simulink model "sampleModel1735"  (R2023a)
settings: Solver=VariableStepAuto  StartTime=0.0  StopTime=10.0  RelTol=1e-3
libraries: hdlsllib x7, simulink x2
settings Model: Creator=user1  LastModifiedBy=user1

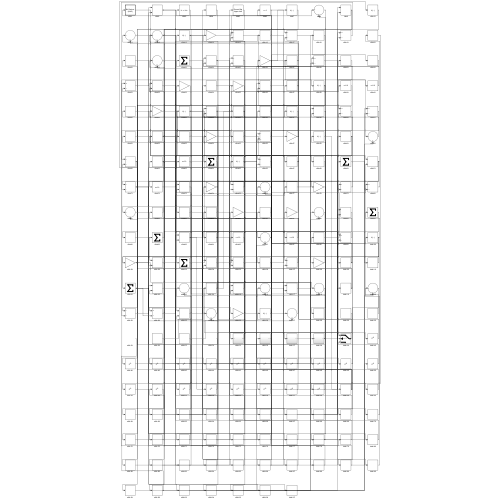
[thumbnail: Simulink's stored preview of the top-level diagram]
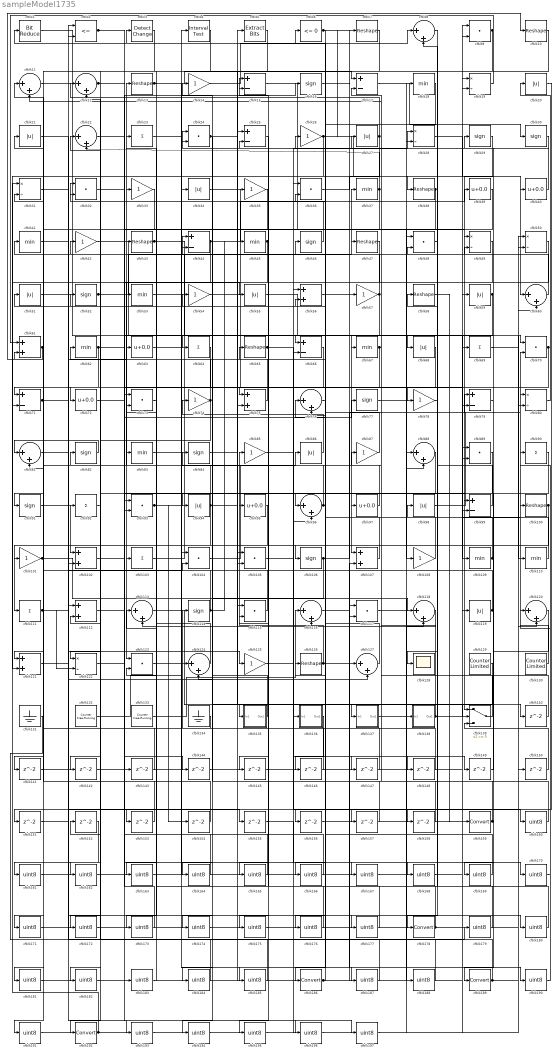
== system sampleModel1735 ==
  cfblk1 : hdlsllib/Logic and Bit Operations/Bit Reduce  mode=AND
  cfblk{7,10,13,38,43,47,58,65,100,126} (10 alike) : Reshape
  cfblk{14,26,33,35,42,54,57,74,78,85,87,101,108,125} (14 alike) : Gain
  cfblk{56,61,75,102,107,112,121} (7 alike) : Sum
  cfblk{23,64,69,90,92,103,111} (7 alike) : Sum  Inputs=+
  cfblk{9,24,32,36,48,70,73,89,93,104..105,115,117,123} (14 alike) : DotProduct  OutDataTypeStr=Inherit: Inherit via internal rule
  cfblk{16,29..30,46,52,77,82,84,91,106,114} (11 alike) : Signum
  cfblk{18,37,41,45,53,62,67,83,109..110} (10 alike) : MinMax
  cfblk{8,11..12,22,60,76,81,88,96,113,116,118,120,124,127} (15 alike) : Sum  Inputs=|++
  cfblk{20..21,27,34,51,55,59,68,86,94,98,119} (12 alike) : Abs  SaturateOnIntegerOverflow=off
  cfblk{19,28,31,49..50,80,122} (7 alike) : Product  Inputs=*/  RndMeth=Zero  SaturateOnIntegerOverflow=on
  cfblk128 : Scope
  cfblk129 : hdlsllib/Sources/Counter Limited  uplimit=7  tsamp=-1
  cfblk130 : hdlsllib/Sources/Counter Limited  uplimit=7  tsamp=-1
  cfblk131 : Ground
  cfblk132 : hdlsllib/Sources/Counter Free-Running  NumBits=16  tsamp=-1
  cfblk133 : hdlsllib/Sources/Counter Free-Running  NumBits=16  tsamp=-1
  cfblk134 : Ground
  cfblk135 : Subsystem
      settings: LibrarySourceBlock=|
      | hdlsllib/Ports &
      | Subsystems/Subsystem
  cfblk136 : Subsystem
      settings: LibrarySourceBlock=|
      | hdlsllib/Ports &
      | Subsystems/Subsystem
  cfblk137 : Subsystem
      settings: LibrarySourceBlock=|
      | hdlsllib/Ports &
      | Subsystems/Subsystem
  cfblk138 : Subsystem
      settings: LibrarySourceBlock=|
      | hdlsllib/Ports &
      | Subsystems/Subsystem
  cfblk139 : Switch  SaturateOnIntegerOverflow=off  InputSameDT=off
  cfblk{140..158} (19 alike) : Delay  SampleTime=1
  cfblk{15,17,25,44,66,71,79,99} (8 alike) : Sum  Inputs=+-
  cfblk{159,178,186,189,192} (5 alike) : DataTypeConversion  SaturateOnIntegerOverflow=off  RndMeth=Floor
  cfblk{160..177,179..185,187..188,190..191,193..197} (34 alike) : DataTypeConversion  OutDataTypeStr=uint8  SaturateOnIntegerOverflow=off  RndMeth=Floor
  cfblk2 : RelationalOperator  Operator=<=  OutDataTypeStr=boolean  InputSameDT=off
  cfblk3 : simulink/Logic and Bit Operations/Detect Change  vinit=0  OutDataTypeStr=boolean
      settings: LibrarySourceBlock=|
      | hdlsllib/Logic and Bit
      | Operations/Detect
      | Change
  cfblk{39..40,63,72,95,97} (6 alike) : Bias  Bias=0.0  SaturateOnIntegerOverflow=off
  cfblk4 : hdlsllib/Logic and Bit Operations/Interval Test  IntervalClosedRight=on  uplimit=0.5  IntervalClosedLeft=on  lowlimit=-0.5  OutDataTypeStr=boolean
  cfblk5 : simulink/Logic and Bit Operations/Extract Bits  bitsToExtract=Upper half  numBits=8  bitIdxRange=[0 7]  outScalingMode=Preserve fixed-point scaling
      settings: LibrarySourceBlock=|
      | hdlsllib/Logic and Bit
      | Operations/Extract Bits
  cfblk6 : hdlsllib/Logic and Bit Operations/Compare To Zero  relop=<=  OutDataTypeStr=boolean
  wires:
  cfblk29/1 -> cfblk139/1
  cfblk34/1 -> cfblk66/1
  cfblk127/1 -> cfblk3/1
  cfblk57/1 -> cfblk37/1, cfblk124/2, cfblk14/1
  cfblk113/1 -> cfblk137/1(In1)
  cfblk82/1 -> cfblk81/1
  cfblk60/1 -> cfblk41/1
  cfblk103/1 -> cfblk46/1
  cfblk15/1 -> cfblk108/1
  cfblk126/1 -> cfblk85/1, cfblk148/1
  cfblk134/1 -> cfblk114/1
  cfblk108/1 -> cfblk82/1
  cfblk43/1 -> cfblk70/1, cfblk117/2
  cfblk109/1 -> cfblk62/1, cfblk8/2
  cfblk74/1 -> cfblk122/1, cfblk12/2
  cfblk130/1 -> cfblk70/2
  cfblk107/1 -> cfblk51/1
  cfblk53/1 -> cfblk124/1
  cfblk96/1 -> cfblk11/1, cfblk56/2
  cfblk64/1 -> cfblk123/1
  cfblk26/1 -> cfblk60/1, cfblk71/2, cfblk7/1
  cfblk123/1 -> cfblk104/1
  cfblk97/1 -> cfblk13/1
  cfblk135/1(Out1) -> cfblk44/1
  cfblk138/1(Out1) -> cfblk100/1, cfblk17/2
  cfblk75/1 -> cfblk33/1
  cfblk87/1 -> cfblk1/1
  cfblk119/1 -> cfblk21/1, cfblk44/2
  cfblk17/1 -> cfblk30/1
  cfblk98/1 -> cfblk80/1
  cfblk12/1 -> cfblk79/2, cfblk196/1
  cfblk88/1 -> cfblk192/1
  cfblk6/1 -> cfblk116/2, cfblk160/1
  cfblk120/1 -> cfblk189/1
  cfblk11/1 -> cfblk110/1
  cfblk51/1 -> cfblk103/1
  cfblk124/1 -> cfblk23/1
  cfblk118/1 -> cfblk113/2
  cfblk54/1 -> cfblk78/1
  cfblk71/1 -> cfblk127/2, cfblk197/1
  cfblk16/1 -> cfblk127/1
  cfblk24/1 -> cfblk118/2, cfblk184/1
  cfblk37/1 -> cfblk72/1, cfblk22/2
  cfblk2/1 -> cfblk49/1, cfblk99/2
  cfblk58/1 -> cfblk159/1
  cfblk99/1 -> cfblk26/1
  cfblk133/1 -> cfblk116/1
  cfblk86/1 -> cfblk74/1
  cfblk80/1 -> cfblk20/1
  cfblk91/1 -> cfblk102/1
  cfblk1/1 -> cfblk107/1
  cfblk79/1 -> cfblk29/1
  cfblk106/1 -> cfblk79/1, cfblk194/1
  cfblk56/1 -> cfblk57/1
  cfblk28/1 -> cfblk40/1
  cfblk38/1 -> cfblk106/1, cfblk64/1
  cfblk39/1 -> cfblk75/1
  cfblk132/1 -> cfblk86/1
  cfblk55/1 -> cfblk109/1
  cfblk22/1 -> cfblk55/1
  cfblk52/1 -> cfblk47/1, cfblk97/1
  cfblk45/1 -> cfblk83/1, cfblk121/1, cfblk15/2
  cfblk42/1 -> cfblk67/1
  cfblk114/1 -> cfblk53/1, cfblk45/1
  cfblk110/1 -> cfblk42/1
  cfblk49/1 -> cfblk135/1(In1)
  cfblk104/1 -> cfblk66/2
  cfblk9/1 -> cfblk91/1, cfblk182/1
  cfblk115/1 -> cfblk95/1
  cfblk139/1 -> cfblk24/1
  cfblk84/1 -> cfblk139/2
  cfblk81/1 -> cfblk63/1
  cfblk8/1 -> cfblk128/1
  cfblk36/1 -> cfblk38/1
  cfblk125/1 -> cfblk56/1
  cfblk101/1 -> cfblk92/1, cfblk138/1(In1)
  cfblk14/1 -> cfblk8/1
  cfblk67/1 -> cfblk94/1, cfblk27/1
  cfblk100/1 -> cfblk111/1, cfblk156/1
  cfblk77/1 -> cfblk18/1
  cfblk46/1 -> cfblk32/1
  cfblk41/1 -> cfblk125/1
  cfblk69/1 -> cfblk80/2
  cfblk76/1 -> cfblk186/1
  cfblk65/1 -> cfblk39/1, cfblk157/1
  cfblk66/1 -> cfblk71/1
  cfblk19/1 -> cfblk61/1
  cfblk47/1 -> cfblk96/1
  cfblk111/1 -> cfblk122/2, cfblk155/1, cfblk177/1
  cfblk31/1 -> cfblk2/2
  cfblk94/1 -> cfblk22/1, cfblk140/1, cfblk141/1
  cfblk92/1 -> cfblk52/1
  cfblk93/1 -> cfblk99/1, cfblk154/1
  cfblk70/1 -> cfblk75/2, cfblk165/1
  cfblk95/1 -> cfblk101/1
  cfblk59/1 -> cfblk93/2, cfblk174/1
  cfblk105/1 -> cfblk28/1
  cfblk40/1 -> cfblk15/1
  cfblk27/1 -> cfblk12/1, cfblk145/1
  cfblk30/1 -> cfblk24/2
  cfblk121/1 -> cfblk104/2
  cfblk13/1 -> cfblk17/1, cfblk118/1, cfblk153/1
  cfblk62/1 -> cfblk68/1, cfblk102/2, cfblk144/1
  cfblk48/1 -> cfblk178/1
  cfblk10/1 -> cfblk105/2
  cfblk72/1 -> cfblk16/1
  cfblk122/1 -> cfblk77/1
  cfblk61/1 -> cfblk10/1, cfblk81/2
  cfblk44/1 -> cfblk9/2, cfblk121/2
  cfblk140/1 -> cfblk11/2
  cfblk141/1 -> cfblk96/2
  cfblk68/1 -> cfblk142/1
  cfblk142/1 -> cfblk9/1
  cfblk102/1 -> cfblk143/1
  cfblk143/1 -> cfblk2/1
  cfblk144/1 -> cfblk28/2
  cfblk145/1 -> cfblk107/2
  cfblk136/1(Out1) -> cfblk146/1
  cfblk146/1 -> cfblk105/1
  cfblk85/1 -> cfblk147/1
  cfblk147/1 -> cfblk31/2
  cfblk148/1 -> cfblk115/2
  cfblk117/1 -> cfblk149/1
  cfblk149/1 -> cfblk49/2
  cfblk150/1 -> cfblk139/3
  cfblk20/1 -> cfblk151/1
  cfblk153/1 -> cfblk32/2
  cfblk154/1 -> cfblk61/2
  cfblk156/1 -> cfblk19/2
  cfblk157/1 -> cfblk6/1
  cfblk78/1 -> cfblk158/1
  cfblk158/1 -> cfblk54/1
  cfblk159/1 -> cfblk87/1, cfblk98/1, cfblk84/1, cfblk65/1
  cfblk160/1 -> cfblk58/1
  cfblk4/1 -> cfblk161/1
  cfblk161/1 -> cfblk34/1
  cfblk7/1 -> cfblk162/1
  cfblk162/1 -> cfblk4/1
  cfblk73/1 -> cfblk163/1
  cfblk163/1 -> cfblk69/1
  cfblk129/1 -> cfblk164/1
  cfblk164/1 -> cfblk73/1
  cfblk165/1 -> cfblk73/2
  cfblk89/1 -> cfblk166/1
  cfblk166/1 -> cfblk115/1
  cfblk63/1 -> cfblk167/1
  cfblk167/1 -> cfblk89/1
  cfblk155/1 -> cfblk168/1
  cfblk168/1 -> cfblk89/2
  cfblk90/1 -> cfblk169/1
  cfblk169/1 -> cfblk36/2
  cfblk32/1 -> cfblk170/1
  cfblk170/1 -> cfblk90/1
  cfblk152/1 -> cfblk171/1
  cfblk171/1 -> cfblk36/1
  cfblk3/1 -> cfblk172/1
  cfblk172/1 -> cfblk152/1
  cfblk5/1 -> cfblk173/1
  cfblk173/1 -> cfblk93/1
  cfblk174/1 -> cfblk5/1
  cfblk25/1 -> cfblk175/1
  cfblk175/1 -> cfblk59/1
  cfblk18/1 -> cfblk176/1
  cfblk176/1 -> cfblk25/1
  cfblk177/1 -> cfblk25/2
  cfblk178/1 -> cfblk60/2, cfblk123/2
  cfblk131/1 -> cfblk179/1
  cfblk179/1 -> cfblk48/1
  cfblk21/1 -> cfblk180/1
  cfblk180/1 -> cfblk48/2
  cfblk35/1 -> cfblk181/1
  cfblk181/1 -> cfblk19/1
  cfblk182/1 -> cfblk35/1
  cfblk112/1 -> cfblk183/1
  cfblk183/1 -> cfblk43/1
  cfblk184/1 -> cfblk112/1
  cfblk83/1 -> cfblk185/1
  cfblk185/1 -> cfblk112/2
  cfblk186/1 -> cfblk117/1, cfblk126/1
  cfblk23/1 -> cfblk187/1
  cfblk187/1 -> cfblk76/1
  cfblk137/1(Out1) -> cfblk188/1
  cfblk188/1 -> cfblk76/2
  cfblk189/1 -> cfblk150/1, cfblk113/1
  cfblk116/1 -> cfblk190/1
  cfblk190/1 -> cfblk120/1
  cfblk33/1 -> cfblk191/1
  cfblk191/1 -> cfblk120/2
  cfblk192/1 -> cfblk119/1, cfblk31/1
  cfblk151/1 -> cfblk193/1
  cfblk193/1 -> cfblk88/1
  cfblk194/1 -> cfblk88/2
  cfblk50/1 -> cfblk195/1
  cfblk195/1 -> cfblk136/1(In1)
  cfblk196/1 -> cfblk50/1
  cfblk197/1 -> cfblk50/2

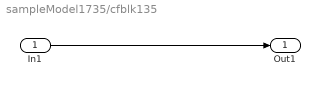
== system sampleModel1735/cfblk135 ==
  In1 : Inport
  Out1 : Outport
  wires:
  In1/1 -> Out1/1

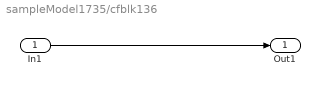
== system sampleModel1735/cfblk136 ==
  In1 : Inport
  Out1 : Outport
  wires:
  In1/1 -> Out1/1

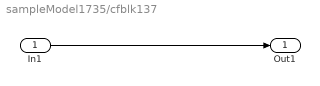
== system sampleModel1735/cfblk137 ==
  In1 : Inport
  Out1 : Outport
  wires:
  In1/1 -> Out1/1

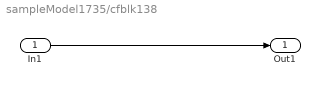
== system sampleModel1735/cfblk138 ==
  In1 : Inport
  Out1 : Outport
  wires:
  In1/1 -> Out1/1
